simulink model "PV_Model_1ststring_shuffle_mppt_2"  (R2019a)
settings: Solver=FixedStepDiscrete  StartTime=0.0  StopTime=1  RelTol=1e-3
libraries: powerlib x27, re_lib x4
settings Model: Creator=burge  LastModifiedBy=natha
settings DataIOCC: SaveState=on  ReturnWorkspaceOutputs=off
settings DebuggingCC: PregeneratedLibrarySubsystemCodeDiagnostic=none  ArithmeticOperatorsInVariantConditions=warning
settings SFSimCC: SimUseLocalCustomCode=off
settings RTWCC: RTWUseLocalCustomCode=off

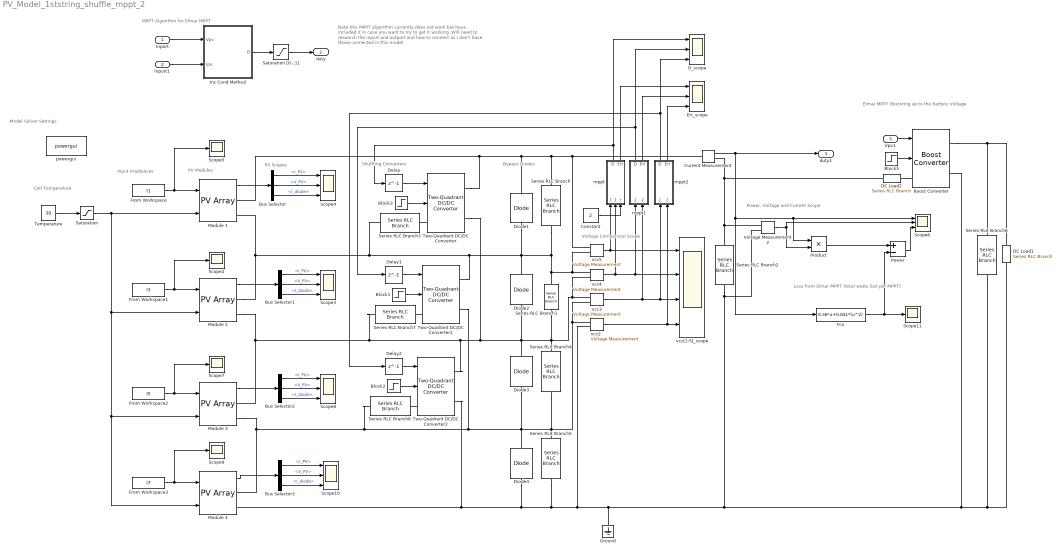
== system PV_Model_1ststring_shuffle_mppt_2 ==
  note: Note this MPPT algorithm currently does not work but have included it in case you want to try to get it working. Will need to research the inport and outport and how to connect as I don't have those connected in this model
  note: Shuffling Converters
  note: PV Modules
  note: Input Irradiances
  note: Model Solver Settings
  note: Cell Temperature
  note: PV Scopes
  note: Bypass Diodes
  note: Voltage Comparison Scope
  note: Elmar MPPT (Boosting up to the
      | Battery Voltage
  note: Power, Voltage and Current
      | Scope
  note: Loss from Elmar MPPT
      | (total watts lost per MPPT)
  note: MPPT Algorithm for Elmar MPPT
  Inport : Inport
  Inport1 : Inport  Port=2
  Vpv1 : Inport  Port=3  OutDataTypeStr=double  PortDimensions=1  SampleTime=[0.0001,0]
  Block1 : Step  Time=0.5  Before=1  After=0  SampleTime=5e-5
  Block2 : Step  Time=0.5  Before=1  After=0  SampleTime=5e-5
  Block3 : Step  Time=0.5  Before=1  After=0  SampleTime=5e-5
  Block5 : Step  Time=0  Before=1  After=0  SampleTime=5e-5
  Boost Converter : powerlib/Power Electronics/Boost Converter  ModelType=Average model (D-controlled)  Ron=1e-3  Rs=1e6  Cs=inf  Vforward=[0,0]  Ron_Diode=1e-3  Rs_Diode=1e6  Cs_Diode=inf  Vf_Diode=1e-3  Rs_CurrentSource=inf
      settings: SourceProductName=Simscape Electrical  SourceProductBaseCode=PS
  Bus Selector{,1..3} (4 alike) : BusSelector  OutputSignals=I_PV,V_PV,I_diode
  Constant : Constant  Value=2
  Current Measurement : powerlib/Measurements/Current Measurement  PhasorSimulation=off  OutputType=Complex  PSBequivalent=0
      settings: SourceProductName=Simscape Electrical
  DC Load1 : powerlib/Elements/Series RLC Branch  LConnTagsString=__new0  RConnTagsString=__new0  BranchType=R  Resistance=9  Inductance=1e-3  SetiL0=off  InitialCurrent=0  Capacitance=1e-6  Setx0=off  InitialVoltage=0  Measurements=None
      settings: SourceProductName=Simscape Electrical
  DC Load2 : powerlib/Elements/Series RLC Branch  LConnTagsString=__new0  RConnTagsString=__new0  BranchType=L  Resistance=9  Inductance=1e-4  SetiL0=off  InitialCurrent=0  Capacitance=1e-6  Setx0=off  InitialVoltage=0  Measurements=None
      settings: SourceProductName=Simscape Electrical
  D_scope : Scope  NumInputPorts=3
  Delay : Delay  DelayLength=1  InitialCondition=0
  Delay1 : Delay  DelayLength=1  InitialCondition=0
  Delay2 : Delay  DelayLength=1  InitialCondition=0
  Diode{1..4} (4 alike) : powerlib/Power Electronics/Diode  Ron=0.05  Lon=0  Vf=0.7  IC=0  UseSnubber=0  Rs=500  Cs=250e-9  Measurements=off
      settings: SourceProductName=Simscape Electrical
  Err_scope : Scope  NumInputPorts=3
  Fcn : Fcn  Expr=0.36*u+0.041*(u^2)
  From Workspace : FromWorkspace  VariableName=I1  OutDataTypeStr=double  SampleTime=0  OutputAfterFinalValue=Holding final value
  From Workspace1 : FromWorkspace  VariableName=I3  OutDataTypeStr=double  SampleTime=0  OutputAfterFinalValue=Holding final value
  From Workspace2 : FromWorkspace  VariableName=I5  OutDataTypeStr=double  SampleTime=0  OutputAfterFinalValue=Holding final value
  From Workspace3 : FromWorkspace  VariableName=I7  OutDataTypeStr=double  SampleTime=0  OutputAfterFinalValue=Holding final value
  Ground : powerlib/Elements/Ground  LConnTagsString=a
      settings: SourceProductName=Simscape Electrical
  Inc Cond Method : Stateflow chart  TreatAsAtomicUnit=on
  Module 1 : re_lib/Solar/PV Array  Npar=1  Nser=5  PlotType=array @ 1000 W/m2 & specified temperatures  S_vec="[ 1000  500  100 ]"  Temp_C_vec="[ 45 25  ]"  ModuleName=User-defined  PlotWhenSelected=off  Pm=3.8912  Ncell=1  Voc=0.727  Isc=6.45  Vm=0.64  Im=6.08  beta_Voc_pc=-0.2393  alpha_Isc_pc=0.045  beta_Voc=-0.0017397  alpha_Isc=0.0029025  IL=6.4807  I0=1.3352e-12  nI=0.96977  Rsh=3.547  Rs=0.00078547  BAL=on  Tc=1e-6  Tfilter=5e-5
      settings: SourceProductName=Simscape Electrical
  Module 2 : re_lib/Solar/PV Array  Npar=1  Nser=10  PlotType=array @ 1000 W/m2 & specified temperatures  S_vec="[ 1000  500  100 ]"  Temp_C_vec="[ 45 25  ]"  ModuleName=User-defined  PlotWhenSelected=off  Pm=3.8912  Ncell=1  Voc=0.727  Isc=6.45  Vm=0.64  Im=6.08  beta_Voc_pc=-0.2393  alpha_Isc_pc=0.045  beta_Voc=-0.0017397  alpha_Isc=0.0029025  IL=6.4807  I0=1.3352e-12  nI=0.96977  Rsh=3.547  Rs=0.00078547  BAL=on  Tc=1e-6  Tfilter=5e-5
      settings: SourceProductName=Simscape Electrical
  Module 3 : re_lib/Solar/PV Array  Npar=1  Nser=10  PlotType=array @ 1000 W/m2 & specified temperatures  S_vec="[ 1000  500  100 ]"  Temp_C_vec="[ 45 25  ]"  ModuleName=User-defined  PlotWhenSelected=off  Pm=3.8912  Ncell=1  Voc=0.727  Isc=6.45  Vm=0.64  Im=6.08  beta_Voc_pc=-0.2393  alpha_Isc_pc=0.045  beta_Voc=-0.0017397  alpha_Isc=0.0029025  IL=6.4807  I0=1.3352e-12  nI=0.96977  Rsh=3.547  Rs=0.00078547  BAL=on  Tc=1e-6  Tfilter=5e-5
      settings: SourceProductName=Simscape Electrical
  Module 4 : re_lib/Solar/PV Array  Npar=1  Nser=10  PlotType=array @ 1000 W/m2 & specified temperatures  S_vec="[ 1000  500  100 ]"  Temp_C_vec="[ 45 25  ]"  ModuleName=User-defined  PlotWhenSelected=off  Pm=3.8912  Ncell=1  Voc=0.727  Isc=6.45  Vm=0.64  Im=6.08  beta_Voc_pc=-0.2393  alpha_Isc_pc=0.045  beta_Voc=-0.0017397  alpha_Isc=0.0029025  IL=6.4807  I0=1.3352e-12  nI=0.96977  Rsh=3.547  Rs=0.00078547  BAL=on  Tc=1e-6  Tfilter=5e-5
      settings: SourceProductName=Simscape Electrical
  Power : Sum  Inputs=+-
  Product : Product
  Saturation : Saturate  UpperLimit=55  LowerLimit=5
  Saturation [0...1] : Saturate  UpperLimit=0.7  LowerLimit=0
  Scope{3..4,6,8,10} (5 alike) : Scope  NumInputPorts=3
  Scope{2,5,7,9,11} (5 alike) : Scope
  Series RLC Branch{,1,4..5} (4 alike) : powerlib/Elements/Series RLC Branch  LConnTagsString=__new0  RConnTagsString=__new0  BranchType=C  Resistance=1  Inductance=1e-3  SetiL0=off  InitialCurrent=0  Capacitance=100e-6  Setx0=off  InitialVoltage=0  Measurements=None
      settings: SourceProductName=Simscape Electrical
  Series RLC Branch2 : powerlib/Elements/Series RLC Branch  LConnTagsString=__new0  RConnTagsString=__new0  BranchType=C  Resistance=1  Inductance=1e-3  SetiL0=off  InitialCurrent=0  Capacitance=10000e-6  Setx0=off  InitialVoltage=0  Measurements=None
      settings: SourceProductName=Simscape Electrical
  Series RLC Branch3 : powerlib/Elements/Series RLC Branch  LConnTagsString=__new0  RConnTagsString=__new0  BranchType=RL  Resistance=0.01  Inductance=1e-4  SetiL0=off  InitialCurrent=0  Capacitance=1e-6  Setx0=off  InitialVoltage=0  Measurements=None
      settings: SourceProductName=Simscape Electrical
  Series RLC Branch6 : powerlib/Elements/Series RLC Branch  LConnTagsString=__new0  RConnTagsString=__new0  BranchType=C  Resistance=1  Inductance=1e-3  SetiL0=off  InitialCurrent=0  Capacitance=10e-6  Setx0=off  InitialVoltage=0  Measurements=None
      settings: SourceProductName=Simscape Electrical
  Series RLC Branch7 : powerlib/Elements/Series RLC Branch  LConnTagsString=__new0  RConnTagsString=__new0  BranchType=RL  Resistance=0.01  Inductance=1e-4  SetiL0=off  InitialCurrent=0  Capacitance=1e-6  Setx0=off  InitialVoltage=0  Measurements=None
      settings: SourceProductName=Simscape Electrical
  Series RLC Branch8 : powerlib/Elements/Series RLC Branch  LConnTagsString=__new0  RConnTagsString=__new0  BranchType=RL  Resistance=0.01  Inductance=1e-4  SetiL0=off  InitialCurrent=0  Capacitance=1e-6  Setx0=off  InitialVoltage=0  Measurements=None
      settings: SourceProductName=Simscape Electrical
  Temperature : Constant  Value=30
  Two-Quadrant DC/DC Converter : powerlib/Power Electronics/Two-Quadrant DC//DC Converter  ModelType=Average model (D-controlled)  Ron=1e-3  Rs=1e6  Cs=inf  Vforward=[0,0]  Ron_Diode=1e-3  Rs_Diode=1e6  Cs_Diode=inf  Vf_Diode=1e-3  Rs_CurrentSource=inf
      settings: SourceProductName=Simscape Electrical  SourceProductBaseCode=PS
  Two-Quadrant DC/DC Converter1 : powerlib/Power Electronics/Two-Quadrant DC//DC Converter  ModelType=Average model (D-controlled)  Ron=1e-3  Rs=1e6  Cs=inf  Vforward=[0,0]  Ron_Diode=1e-3  Rs_Diode=1e6  Cs_Diode=inf  Vf_Diode=1e-3  Rs_CurrentSource=inf
      settings: SourceProductName=Simscape Electrical  SourceProductBaseCode=PS
  Two-Quadrant DC/DC Converter2 : powerlib/Power Electronics/Two-Quadrant DC//DC Converter  ModelType=Average model (D-controlled)  Ron=1e-3  Rs=1e6  Cs=inf  Vforward=[0,0]  Ron_Diode=1e-3  Rs_Diode=1e6  Cs_Diode=inf  Vf_Diode=1e-3  Rs_CurrentSource=inf
      settings: SourceProductName=Simscape Electrical  SourceProductBaseCode=PS
  Voltage Measurement2 : powerlib/Measurements/Voltage Measurement  PhasorSimulation=off  OutputType=Complex  PSBequivalent=0
      settings: SourceProductName=Simscape Electrical
  mppt : Subsystem
  mppt1 : Subsystem
  mppt2 : Subsystem
  powergui : powerlib/powergui  Priority=1  SimulationMode=Discrete  SampleTime=5e-6  frequency=60  Iterations=50  frequencyindice=0  Pbase=100e6  ErrMax=1e-4  UnitsV=kV  UnitsW=MW  buscounter=0  FunctionMessages=off  echomessages=off  EnableUseOfTLC=off  CurrentSourceSwitches=off  DisableSnubberDevices=off  DisableRonSwitches=off  DisableVfSwitches=off  DisplayEquations=off  AutomaticDiscreteSolvers=off  SolverType=Tustin/Backward Euler (TBE)  Interpol=off  ExternalGateDelay=off  methode=off  Ts=100  x0status=blocks  SPID=off  SwTol=0  HookPort=off  NonlinearTolerance=0  nMaxIteration=15  ContinueOnMaxIteration=off  RestoreLinks=warning  ResistiveCurrentMeasurement=off  Frange=[0:2:500]  Ylog=off  Xlog=on  ShowGrid=off  save=off  variable=ZData  structure=0  ZoomFFT=off  StartTime=0.0  cycles=1  DisplayStyle=1  fundamental=60  FreqAxis=off  MaxFrequency=1000  frequencyindicesteady=1  RmsSteady=1  display=off
      settings: SourceProductName=Simscape Electrical
  vcc{2..5} (4 alike) : powerlib/Measurements/Voltage Measurement  PhasorSimulation=off  OutputType=Complex  PSBequivalent=0
      settings: SourceProductName=Simscape Electrical
  vcc[2:5]_scope : Scope  NumInputPorts=4
  duty1 : Outport  OutDataTypeStr=double  PortDimensions=1  SampleTime=[0.0001,0]
  duty : Outport  Port=2  OutDataTypeStr=double  PortDimensions=1  SampleTime=[0.0001,0]
  wires:
  Module 1/1 -> Bus Selector/1
  Bus Selector/1 -> Scope4/1  "<I_PV>"
  From Workspace/1 -> Scope5/1, Module 1/1
  Temperature/1 -> Saturation/1
  Bus Selector/2 -> Scope4/2  "<V_PV>"
  Bus Selector/3 -> Scope4/3  "<I_diode>"
  vcc5/1 -> mppt/1(Vin1), vcc[2:5]_scope/1
  Saturation/1 -> Module 4/2, Module 3/2, Module 2/2, Module 1/2
  From Workspace1/1 -> Scope2/1, Module 2/1
  Bus Selector1/2 -> Scope3/2  "<V_PV>"
  Bus Selector1/3 -> Scope3/3  "<I_diode>"
  Module 2/1 -> Bus Selector1/1
  Bus Selector1/1 -> Scope3/1  "<I_PV>"
  vcc4/1 -> mppt1/1(Vin1), vcc[2:5]_scope/2, mppt/2(Vin2)
  From Workspace2/1 -> Scope7/1, Module 3/1
  Bus Selector2/1 -> Scope8/1  "<I_PV>"
  Bus Selector2/3 -> Scope8/3  "<I_diode>"
  Bus Selector2/2 -> Scope8/2  "<V_PV>"
  Module 3/1 -> Bus Selector2/1
  vcc3/1 -> mppt1/2(Vin2), mppt2/1(Vin1), vcc[2:5]_scope/3
  From Workspace3/1 -> Scope9/1, Module 4/1
  Bus Selector3/2 -> Scope10/2  "<V_PV>"
  Bus Selector3/1 -> Scope10/1  "<I_PV>"
  Bus Selector3/3 -> Scope10/3  "<I_diode>"
  Module 4/1 -> Bus Selector3/1
  vcc2/1 -> mppt2/2(Vin2), vcc[2:5]_scope/4
  Block1/1 -> Two-Quadrant DC/DC Converter1/2
  Block2/1 -> Two-Quadrant DC/DC Converter2/2
  Delay2/1 -> Two-Quadrant DC/DC Converter2/1
  Block5/1 -> Boost Converter/2
  Inc Cond Method/1(D) -> Saturation [0...1]/1
  Saturation [0...1]/1 -> duty/1
  Product/1 -> Power/1
  Fcn/1 -> Power/2, Scope11/1
  Power/1 -> Scope6/3
  Vpv1/1 -> Boost Converter/1
  Current Measurement/1 -> Fcn/1, Product/1, Scope6/1, duty1/1
  Voltage Measurement2/1 -> Scope6/2, Product/2
  Delay1/1 -> Two-Quadrant DC/DC Converter1/1
  mppt/1(D) -> Delay/1, D_scope/1
  Delay/1 -> Two-Quadrant DC/DC Converter/1
  mppt1/1(D) -> D_scope/2, Delay1/1
  mppt2/1(D) -> D_scope/3, Delay2/1
  mppt/2(Err) -> Err_scope/1
  mppt1/2(Err) -> Err_scope/2
  mppt2/2(Err) -> Err_scope/3
  Constant/1 -> mppt/3(r)
  Inport/1 -> Inc Cond Method/1(Vpv)
  Inport1/1 -> Inc Cond Method/2(Ipv)
  Block3/1 -> Two-Quadrant DC/DC Converter/2
  connections:
  Voltage Measurement2/LConn1 -- DC Load2/LConn1 -- Current Measurement/RConn1 -- Series RLC Branch2/LConn1
  Series RLC Branch3/RConn1 -- Two-Quadrant DC/DC Converter/LConn1
  Module 2/RConn2 -- Module 3/RConn1 -- Series RLC Branch7/LConn1 -- Two-Quadrant DC/DC Converter2/RConn1 -- Two-Quadrant DC/DC Converter/RConn2 -- Series RLC Branch1/RConn1 -- vcc3/LConn1 -- vcc4/LConn2 -- Series RLC Branch4/LConn1 -- Diode2/LConn1 -- Diode3/RConn1
  Series RLC Branch4/RConn1 -- Series RLC Branch5/LConn1 -- vcc3/LConn2 -- vcc2/LConn1 -- Diode4/RConn1 -- Diode3/LConn1 -- Two-Quadrant DC/DC Converter1/RConn2 -- Module 4/RConn1 -- Module 3/RConn2 -- Series RLC Branch8/LConn1
  Series RLC Branch/LConn1 -- Diode1/RConn1 -- Two-Quadrant DC/DC Converter/RConn1 -- Module 1/RConn1 -- Current Measurement/LConn1 -- vcc5/LConn1
  Series RLC Branch7/RConn1 -- Two-Quadrant DC/DC Converter1/LConn1
  Series RLC Branch8/RConn1 -- Two-Quadrant DC/DC Converter2/LConn1
  Voltage Measurement2/LConn2 -- Ground/LConn1 -- vcc2/LConn2 -- Series RLC Branch5/RConn1 -- Two-Quadrant DC/DC Converter2/RConn2 -- Module 4/RConn2 -- Diode4/LConn1 -- Boost Converter/RConn2 -- Series RLC Branch6/RConn1 -- DC Load1/RConn1 -- Series RLC Branch2/RConn1
  Boost Converter/RConn1 -- Series RLC Branch6/LConn1 -- DC Load1/LConn1
  DC Load2/RConn1 -- Boost Converter/LConn1
  Module 2/RConn1 -- Series RLC Branch3/LConn1 -- Two-Quadrant DC/DC Converter1/RConn1 -- Diode2/RConn1 -- Diode1/LConn1 -- Series RLC Branch/RConn1 -- vcc5/LConn2 -- vcc4/LConn1 -- Series RLC Branch1/LConn1 -- Module 1/RConn2

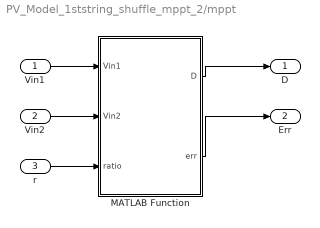
== system PV_Model_1ststring_shuffle_mppt_2/mppt ==
  Vin1 : Inport
  Vin2 : Inport  Port=2
  r : Inport  Port=3
  MATLAB Function : MATLAB Function  TreatAsAtomicUnit=on
  D : Outport
  Err : Outport  Port=2
  wires:
  Vin1/1 -> MATLAB Function/1(Vin1)
  Vin2/1 -> MATLAB Function/2(Vin2)
  MATLAB Function/1(D) -> D/1
  MATLAB Function/2(err) -> Err/1
  r/1 -> MATLAB Function/3(ratio)

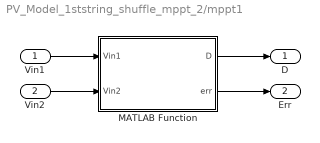
== system PV_Model_1ststring_shuffle_mppt_2/mppt1 ==
  Vin1 : Inport
  Vin2 : Inport  Port=2
  MATLAB Function : MATLAB Function  TreatAsAtomicUnit=on
  D : Outport
  Err : Outport  Port=2
  wires:
  Vin1/1 -> MATLAB Function/1(Vin1)
  Vin2/1 -> MATLAB Function/2(Vin2)
  MATLAB Function/1(D) -> D/1
  MATLAB Function/2(err) -> Err/1

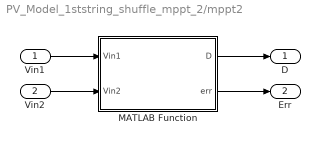
== system PV_Model_1ststring_shuffle_mppt_2/mppt2 ==
  Vin1 : Inport
  Vin2 : Inport  Port=2
  MATLAB Function : MATLAB Function  TreatAsAtomicUnit=on
  D : Outport
  Err : Outport  Port=2
  wires:
  Vin1/1 -> MATLAB Function/1(Vin1)
  Vin2/1 -> MATLAB Function/2(Vin2)
  MATLAB Function/1(D) -> D/1
  MATLAB Function/2(err) -> Err/1

== stateflow chart PV_Model_1ststring_shuffle_mppt_2/Inc Cond Method ==
  settings: updateMethod=DISCRETE  sampleTime=1e-4
  state SAMPLEandCALCULATE
    entry:
    deltaV = Vpv - Vprev;
    deltaI = Ipv - Iprev;
    d = D;
  state INCREMENT_DUTY
    entry:
    d = d + deltad;
  state DECREMENT_DUTY
    entry:
    d = d - deltad;
  state RETURN
    entry:
    Vprev = Vpv; Iprev = Ipv;
    D = d;
  (default) -> SAMPLEandCALCULATE
  RETURN -> SAMPLEandCALCULATE
  SAMPLEandCALCULATE -> (junction 14) [order 1] : [deltaV > Vtol || deltaV < -Vtol]
  SAMPLEandCALCULATE -> (junction 15) [order 2]
  (junction 15) -> RETURN [order 3]
  (junction 15) -> INCREMENT_DUTY [order 1] : [deltaI < -Itol]
  (junction 14) -> RETURN [order 3]
  (junction 14) -> DECREMENT_DUTY [order 1] : [deltaI/deltaV > -Ipv/Vpv]
  (junction 14) -> INCREMENT_DUTY [order 2] : [deltaI/deltaV < -Ipv/Vpv]
  (junction 15) -> DECREMENT_DUTY [order 2] : [deltaI > Itol]
  INCREMENT_DUTY -> RETURN
  DECREMENT_DUTY -> RETURN
  data: Vpv input; Ipv input; D output double =0.67; Vprev local double =0; Iprev local double =0; Itol constant double =0.001; Vtol constant double =0.001; deltad constant double =0.0025; deltaV local double =0; deltaI local double =0; d local double =0

== matlab function PV_Model_1ststring_shuffle_mppt_2/mppt1/MATLAB Function ==
  data: Vin1 input; D output; Vin2 input; err output
function [D,err] = getD(Vin1, Vin2)

% Increase in D => decrease in Vin1

err = Vin1 - Vin2;

Vin = Vin1 + Vin2;
Vout = Vin1;

D = Vout/Vin;

if (D > 0) && (D < 1) % If valid
    if (err > 0) % if Vin1 > Vin2
        D = D + 0.001;
    elseif (err < 0) % Vin1 < Vin2
        D = D - 0.001;
    end
elseif D > 1 % set upper lim to 1
    D = 1;
elseif D < 0 % Set lower lim to 0
    D = 0;
end

== matlab function PV_Model_1ststring_shuffle_mppt_2/mppt2/MATLAB Function ==
  data: Vin1 input; D output; Vin2 input; err output
function [D,err] = getD(Vin1, Vin2)

% Increase in D => decrease in Vin1

err = Vin1 - Vin2;

Vin = Vin1 + Vin2;
Vout = Vin1;

D = Vout/Vin;

if (D > 0) && (D < 1) % If valid
    if (err > 0) % if Vin1 > Vin2
        D = D + 0.001;
    elseif (err < 0) % Vin1 < Vin2
        D = D - 0.001;
    end
elseif D > 1 % set upper lim to 1
    D = 1;
elseif D < 0 % Set lower lim to 0
    D = 0;
end

== matlab function PV_Model_1ststring_shuffle_mppt_2/mppt/MATLAB Function ==
  data: Vin1 input; D output; Vin2 input; err output; ratio input
function [D, err] = getD(Vin1, Vin2, ratio)

% Increase in D => decrease in Vin1
%               => increase in Vin2
if (abs(Vin1) == 0) ||  (abs(Vin2) == 0)
    shdn = 1;
else
    shdn = 0;
end


Kp = 1;

err = ratio*Vin1 - Vin2;

Vin = ratio*Vin1 + Vin2;
Vout = Vin1;
% Calculate old D
D = Vout/Vin;

if (D > 0) && (D < 1) % If valid
%     if (err > 0) % if Vin1 > Vin2
%         D = D + 0.001;
%     elseif (err < 0) % Vin1 < Vin2
%         D = D - 0.001;
%     end
    D = D + Kp*err;
elseif D > 1 % set upper lim to 1
    D = 1;
elseif D < 0 % Set lower lim to 0
    D = 0;
end
